simulink model "computed_torque_control"  (R2015a)
settings: Solver=ode45  StartTime=0.0  StopTime=10  RelTol=1e-3
settings Model: Creator=admin  LastModifiedBy=admin

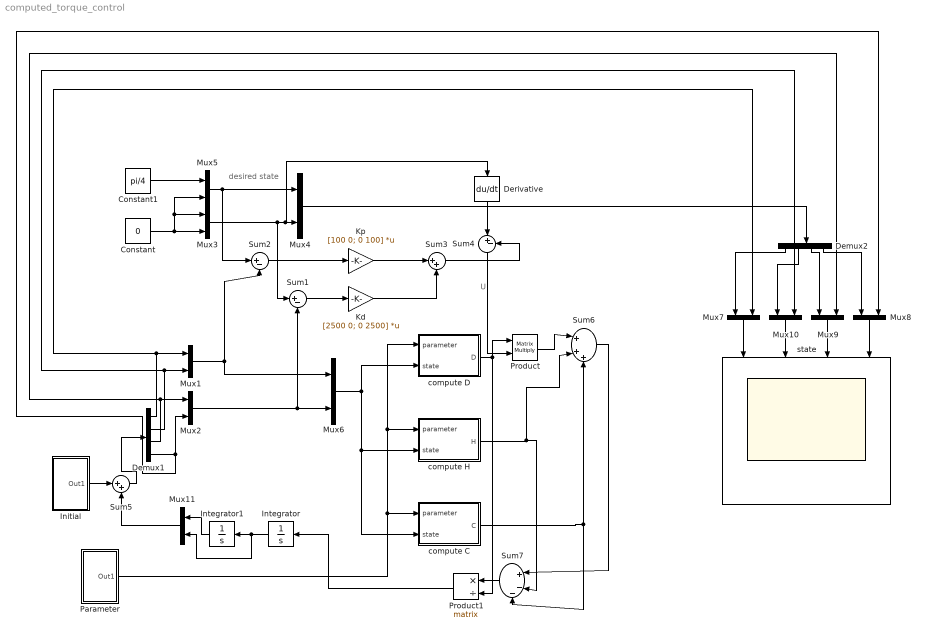
== system computed_torque_control ==
  note: U
  note: desired state
  Constant : Constant  Value=0
  Constant1 : Constant  Value=pi/4
  Demux1 : Demux
  Demux2 : Demux
  Derivative : Derivative
  Initial : Subsystem
  Integrator : Integrator
  Integrator1 : Integrator
  Kd : Gain  Gain=[2500 0; 0 2500]  Multiplication=Matrix(K*u)
  Kp : Gain  Gain=[100 0; 0 100]  Multiplication=Matrix(K*u)
  Mux{1..11} (11 alike) : Mux  Inputs=2
  Parameter : Subsystem
  Product : Product  Inputs=**  Multiplication=Matrix(*)
  Product1 : Product  Inputs=*/  Multiplication=Matrix(*)
  Sum1 : Sum  Inputs=|+-
  Sum2 : Sum  Inputs=|+-
  Sum3 : Sum  Inputs=|++
  Sum4 : Sum  Inputs=|+-
  Sum5 : Sum  Inputs=|++
  Sum6 : Sum  Inputs=|+++
  Sum7 : Sum  Inputs=|+--
  compute C : MATLAB Function  TreatAsAtomicUnit=on
  compute D : MATLAB Function  TreatAsAtomicUnit=on
  compute H : MATLAB Function  TreatAsAtomicUnit=on
  "state " : Scope  NumInputPorts=4
      settings: YMin=-5~-5~-5~-5  YMax=5~5~5~5
  wires:
  Constant1/1 -> Mux5/1
  Constant/1 -> Mux3/2, Mux3/1, Mux5/2
  Mux4/1 -> Demux2/1
  Initial/1(Out1) -> Sum5/1
  Parameter/1(Out1) -> compute D/1(parameter), compute H/1(parameter), compute C/1(parameter)
  compute D/1(D) -> Product1/2, Product/1
  Mux1/1 -> Mux6/1, Sum2/2
  Mux5/1 -> Sum2/1, Mux4/1
  Mux3/1 -> Derivative/1, Mux4/2, Sum1/1
  Mux2/1 -> Mux6/2, Sum1/2
  Sum2/1 -> Kp/1
  Sum1/1 -> Kd/1
  Kp/1 -> Sum3/1
  Kd/1 -> Sum3/2
  Sum3/1 -> Sum4/2
  Mux6/1 -> compute D/2(state), compute C/2(state), compute H/2(state)
  compute H/1(H) -> Sum7/2, Sum6/2
  compute C/1(C) -> Sum7/3, Sum6/3
  Mux7/1 -> "state "/1
  Mux10/1 -> "state "/2
  Mux9/1 -> "state "/3
  Mux8/1 -> "state "/4
  Demux2/1 -> Mux7/1
  Demux2/2 -> Mux10/1
  Demux2/3 -> Mux9/1
  Demux2/4 -> Mux8/1
  Demux1/1 -> Mux7/2, Mux1/1
  Demux1/2 -> Mux10/2, Mux1/2
  Demux1/3 -> Mux2/1, Mux9/2
  Demux1/4 -> Mux2/2, Mux8/2
  Derivative/1 -> Sum4/1
  Product/1 -> Sum6/1
  Sum6/1 -> Sum7/1
  Sum7/1 -> Product1/1
  Sum4/1 -> Product/2
  Product1/1 -> Integrator/1
  Integrator/1 -> Mux11/2, Integrator1/1
  Mux11/1 -> Sum5/2
  Sum5/1 -> Demux1/1
  Integrator1/1 -> Mux11/1

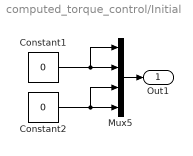
== system computed_torque_control/Initial ==
  Constant1 : Constant  Value=0
  Constant2 : Constant  Value=0
  Mux5 : Mux
  Out1 : Outport
  wires:
  Constant1/1 -> Mux5/1, Mux5/2
  Mux5/1 -> Out1/1
  Constant2/1 -> Mux5/4, Mux5/3

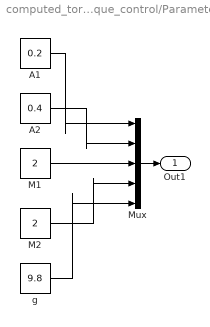
== system computed_torque_control/Parameter ==
  A1 : Constant  Value=0.2
  A2 : Constant  Value=0.4
  M1 : Constant  Value=2
  M2 : Constant  Value=2
  Mux : Mux  Inputs=5
  g : Constant  Value=9.8
  Out1 : Outport
  wires:
  A1/1 -> Mux/1
  g/1 -> Mux/5
  M1/1 -> Mux/3
  Mux/1 -> Out1/1
  A2/1 -> Mux/2
  M2/1 -> Mux/4

== matlab function computed_torque_control/compute H ==
  data: parameter input; H output; state input
function H = H(parameter,state)
a1 = parameter(1);
a2 = parameter(2);
m1 = parameter(3);
m2 = parameter(4);
g = parameter(5);

if isempty(state)
    th1 = 0;
    th2 = 0;
    thd1 = 0;
    thd2 = 0;
else
    th1 = state(1);
    th2 = state(2);
    thd1 = state(3);
    thd2 = state(4);
end
H = [ -(a1*a2*m2*thd2*sin(th2)*(2*thd1 + thd2))/2;
                (a1*a2*m2*thd1^2*sin(th2))/2];

== matlab function computed_torque_control/compute D ==
  data: parameter input; D output; state input
function D = D(parameter,state)
a1 = parameter(1);
a2 = parameter(2);
m1 = parameter(3);
m2 = parameter(4);
g = parameter(5);

if isempty(state)
    th1 = 0;
    th2 = 0;
    thd1 = 0;
    thd2 = 0;
else
    th1 = state(1);
    th2 = state(2);
    thd1 = state(3);
    thd2 = state(4);
end

D = [ (a1^2*m1)/3 + a1^2*m2 + (a2^2*m2)/3 + a1*a2*m2*cos(th2), (a2*m2*(2*a2 + 3*a1*cos(th2)))/6;
    (a2*m2*(2*a2 + 3*a1*cos(th2)))/6,                      (a2^2*m2)/3];

== matlab function computed_torque_control/compute C ==
  data: parameter input; C output; state input
function C = C(parameter,state)
a1 = parameter(1);
a2 = parameter(2);
m1 = parameter(3);
m2 = parameter(4);
g = parameter(5);
if isempty(state)
    th1 = 0;
    th2 = 0;
    thd1 = 0;
    thd2 = 0;
else
    th1 = state(1);
    th2 = state(2);
    thd1 = state(3);
    thd2 = state(4);
end
C = [(g*(a1*m1*cos(th1) + 2*a1*m2*cos(th1) + a2*m2*cos(th1 + th2)))/2;
                                       (a2*g*m2*cos(th1 + th2))/2];
